simulink model "cubesat_attitude"  (R2025b)
settings: Solver=VariableStepAuto  StartTime=0.0  StopTime=20  RelTol=1e-3
values from neighbouring files (symbols this model uses):
  Izz = (1/12) * mass * (width^2 + height^2)    (= 0.00666666666667)    [init_attitude.m]
  Kd = 0.0107    [init_attitude.m]
  Kp = 0.0067    [init_attitude.m]
  omega0 = 0    [init_attitude.m]
  tau_max = 0.002    [init_attitude.m]
  theta0 = deg2rad(30)    [init_attitude.m]
  theta_cmd = 0    [init_attitude.m]
settings Model: Creator=matho  LastModifiedBy=matho

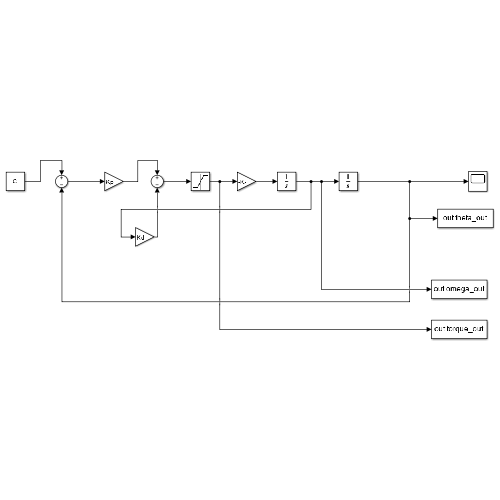
[thumbnail: Simulink's stored preview of the top-level diagram]
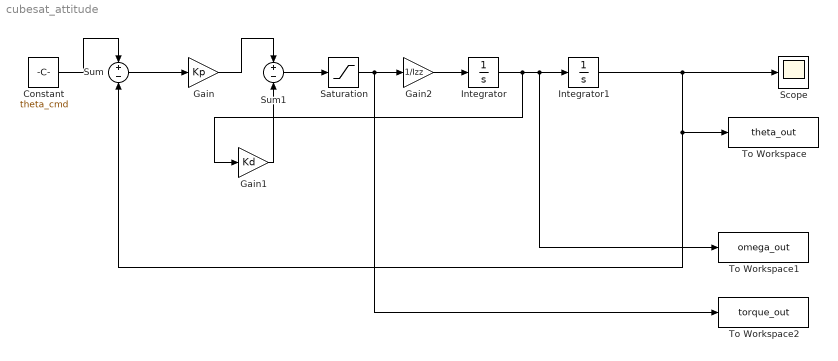
== system cubesat_attitude ==
  Constant : Constant  Value=theta_cmd
  Gain : Gain  Gain=Kp
  Gain1 : Gain  Gain=Kd
  Gain2 : Gain  Gain=1/Izz
  Integrator : Integrator  InitialCondition=omega0
  Integrator1 : Integrator  InitialCondition=theta0
  Saturation : Saturate  UpperLimit=tau_max  LowerLimit=-tau_max
  Scope : Scope
      settings: ActiveDisplayYMinimum=-0.10561803482511284  ActiveDisplayYMaximum=0.62664292038152847
  Sum : Sum  Inputs=+-
  Sum1 : Sum  Inputs=+-
  To Workspace : ToWorkspace  VariableName=theta_out  SaveFormat=Timeseries  SampleTime=-1
  To Workspace1 : ToWorkspace  VariableName=omega_out  SaveFormat=Timeseries  SampleTime=-1
  To Workspace2 : ToWorkspace  VariableName=torque_out  SaveFormat=Timeseries  SampleTime=-1
  wires:
  Constant/1 -> Sum/1
  Sum/1 -> Gain/1
  Gain/1 -> Sum1/1
  Sum1/1 -> Saturation/1
  Saturation/1 -> To Workspace2/1, Gain2/1
  Gain2/1 -> Integrator/1
  Gain1/1 -> Sum1/2
  Integrator/1 -> Gain1/1, To Workspace1/1, Integrator1/1
  Integrator1/1 -> Scope/1, Sum/2, To Workspace/1
